simulink model "CCACC_DESIGN"  (R2023b)
settings: Solver=VariableStepAuto  StartTime=0.0  StopTime=200  RelTol=1e-3
values from neighbouring files (symbols this model uses):
  plant_den = [1084 17]    [CCACCDESIGN.m]
  plant_num = 1    [CCACCDESIGN.m]
  V_set_speed = str2double(answer)    [CCACCDESIGN.m]
undefined symbols (not defined in the file or in its folder): sigbuilder_block
libraries: slpidlib x1
settings Model: Creator=ADEL  LastModifiedBy=ADEL

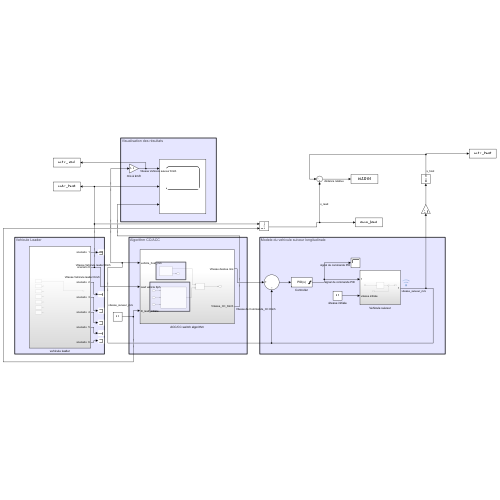
[thumbnail: Simulink's stored preview of the top-level diagram]
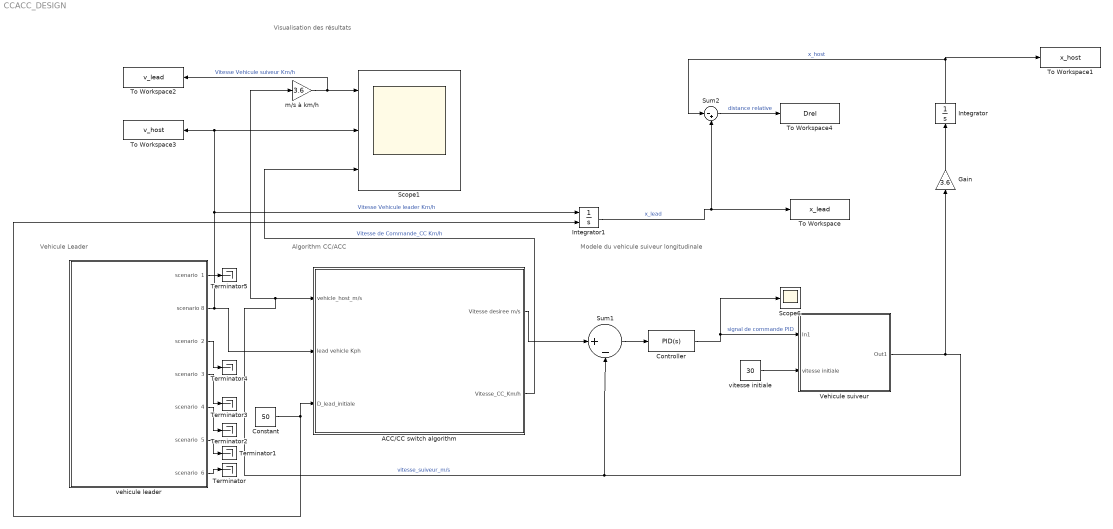
== system CCACC_DESIGN ==
  note: Visualisation des résultats
  note: Vehicule Leader
  note: Algorithm CC/ACC
  note: Modele du vehicule suiveur longitudinale
  ACC/CC switch algorithm : Subsystem
  Constant : Constant  Value=50
  Controller : slpidlib/PID Controller  Controller=PID  Form=Parallel  TimeDomain=Continuous-time  UseExternalTs=off  SampleTime=-1  IntegratorMethod=Forward Euler  FilterMethod=Forward Euler  ControllerParametersSource=internal  P=142.14884257668  I=6.71648983660147  UseKiTs=off  D=262.976834722354  N=0.25  UseFilter=on  TunerSelectOption=Transfer Function Based (PID Tuner App)  InitialConditionSource=internal  InitialConditionForIntegrator=0  InitialConditionForFilter=0  DifferentiatorICPrevScaledInput=0  ExternalReset=none  TrackingMode=off  Kt=1  LimitOutput=on  SatLimitsSource=internal  UpperSaturationLimit=4600  LowerSaturationLimit=-4600  LinearizeAsGain=on  AntiWindupMode=none  Kb=1  LimitIntegrator=off  UpperIntegratorSaturationLimit=inf  LowerIntegratorSaturationLimit=-inf  POutMin=[]  POutMax=[]  IOutMin=[]  IOutMax=[]  DOutMin=[]  DOutMax=[]  NOutMin=[]  NOutMax=[]  SumOutMin=[]  SumOutMax=[]  SaturationOutMin=[]  SaturationOutMax=[]  PParamMin=[]  PParamMax=[]  IParamMin=[]  IParamMax=[]  DParamMin=[]  DParamMax=[]  NParamMin=[]  NParamMax=[]  KbParamMin=[]  KbParamMax=[]  KtParamMin=[]  KtParamMax=[]  KbOutMin=[]  KbOutMax=[]  KtOutMin=[]  KtOutMax=[]  IntegratorOutMin=[]  IntegratorOutMax=[]  FilterOutMin=[]  FilterOutMax=[]  SumI1OutMin=[]  SumI1OutMax=[]  SumI2OutMin=[]  SumI2OutMax=[]  SumI3OutMin=[]  SumI3OutMax=[]  SumI4OutMin=[]  SumI4OutMax=[]  SumDOutMin=[]  SumDOutMax=[]  DifferentiatorOutMin=[]  DifferentiatorOutMax=[]  FilterDiffOutCoefMin=[]  FilterDiffOutCoefMax=[]  ReciprocalOutMin=[]  ReciprocalOutMax=[]  SumDenOutMin=[]  SumDenOutMax=[]  SumNumOutMin=[]  SumNumOutMax=[]  DivideOutMin=[]  DivideOutMax=[]  UdiffTsProdOutMin=[]  UdiffTsProdOutMax=[]  NTsProdOutMin=[]  NTsProdOutMax=[]  UintegralTsProdOutMin=[]  UintegralTsProdOutMax=[]  UngainTsProdOutMin=[]  UngainTsProdOutMax=[]  ClampingZeroOutDataTypeStr=Inherit: Inherit via back propagation  ClampingZeroOutMin=[]  ClampingZeroOutMax=[]  FilterDenConstantOutDataTypeStr=Inherit: Inherit via back propagation  FilterDenConstantOutMin=[]  FilterDenConstantOutMax=[]  PCopyOutDataTypeStr=Inherit: Inherit via back propagation  PCopyOutMin=[]  PCopyOutMax=[]  NCopyOutDataTypeStr=Inherit: Inherit via back propagation  NCopyOutMin=[]  NCopyOutMax=[]  IntegratorContinuousStateAttributes=''  IntegratorStateMustResolveToSignalObject=off  IntegratorRTWStateStorageClass=Auto  FilterContinuousStateAttributes=''  FilterStateMustResolveToSignalObject=off  FilterRTWStateStorageClass=Auto  ParallelPVariant=InternalParameters  IdealPVariant=Disabled  IVariant=InternalParameters  DVariant=InternalParameters  IntegratorVariant=Continuous  SatVariant=Enabled  AWVariant=Passthrough  PCopyVariant=Disabled  TRVariant=Disabled  FdbkBlocksVariant=Forward  IdealPFdbkVariant=Disabled  SatFdbkVariant=Disabled  DerivativeFilterVariant=ContFilter  NVariant=InternalParameters  NCopyVariant=Disabled  FilterICVariant=InternalICsFilter  IntegratorICVariant=InternalICs  ExternalResetVariant=Disabled  TRSumVariant=Passthrough  SumFdbkVariant=Disabled  SumVariant=Sum_PID  TsampFilterVariant=InternalTs  TsampNgainVariant=Passthrough  TsampIntegralVariant=Disabled_SignalSpec  ExternalSaturationOutDataTypeStr=Inherit: Same as second input
  Gain : Gain  Gain=3.6
  Integrator : Integrator
  Integrator1 : Integrator  InitialConditionSource=external  InitialCondition=50
  Scope1 : Scope  NumInputPorts=3
  Scope6 : Scope
  Sum1 : Sum  Inputs=|+-
  Sum2 : Sum  Inputs=|-+
  Terminator{,1..5} (6 alike) : Terminator
  To Workspace : ToWorkspace  VariableName=x_lead  SaveFormat=Structure With Time  SampleTime=-1
  To Workspace1 : ToWorkspace  VariableName=x_host  SaveFormat=Structure With Time  SampleTime=-1
  To Workspace2 : ToWorkspace  VariableName=v_lead  SaveFormat=Structure With Time  SampleTime=-1
  To Workspace3 : ToWorkspace  VariableName=v_host  SaveFormat=Structure With Time  SampleTime=-1
  To Workspace4 : ToWorkspace  VariableName=Drel  SaveFormat=Structure With Time  SampleTime=-1
  Vehicule suiveur : Subsystem
  m/s à km/h : Gain  Gain=3.6
  vehicule leader : Subsystem
  vitesse initiale : Constant  Value=30
  wires:
  Gain/1 -> Integrator/1
  vehicule leader/3(scenario  2) -> Terminator4/1
  Constant/1 -> ACC/CC switch algorithm/3(D_lead_initiale), Integrator1/2
  vehicule leader/4(scenario  3) -> Terminator3/1
  vitesse initiale/1 -> Vehicule suiveur/2(vitesse initiale)
  vehicule leader/7(scenario  6) -> Terminator/1
  Sum2/1 -> To Workspace4/1  "distance relative"
  Controller/1 -> Scope6/1, Vehicule suiveur/1(In1)  "signal de commande PID"
  vehicule leader/1(scenario  1) -> Terminator5/1
  Integrator/1 -> To Workspace1/1, Sum2/1  "x_host"
  vehicule leader/5(scenario  4) -> Terminator2/1
  Vehicule suiveur/1(Out1) -> ACC/CC switch algorithm/1(vehicle_host_m/s), m/s à km/h/1, Sum1/2, Gain/1  "vitesse_suiveur_m/s"
  vehicule leader/2(scenario 8) -> To Workspace3/1, Scope1/2, Integrator1/1, ACC/CC switch algorithm/2(lead vehicle Kph)  "Vitesse Vehicule leader Km/h"
  vehicule leader/6(scenario  5) -> Terminator1/1
  ACC/CC switch algorithm/2(Vitesse_CC_Km/h) -> Scope1/3  "Vitesse de Commande_CC Km/h"
  m/s à km/h/1 -> To Workspace2/1, Scope1/1  "Vitesse Vehicule suiveur Km/h"
  Integrator1/1 -> Sum2/2, To Workspace/1  "x_lead"
  Sum1/1 -> Controller/1
  ACC/CC switch algorithm/1(Vitesse desiree m/s) -> Sum1/1

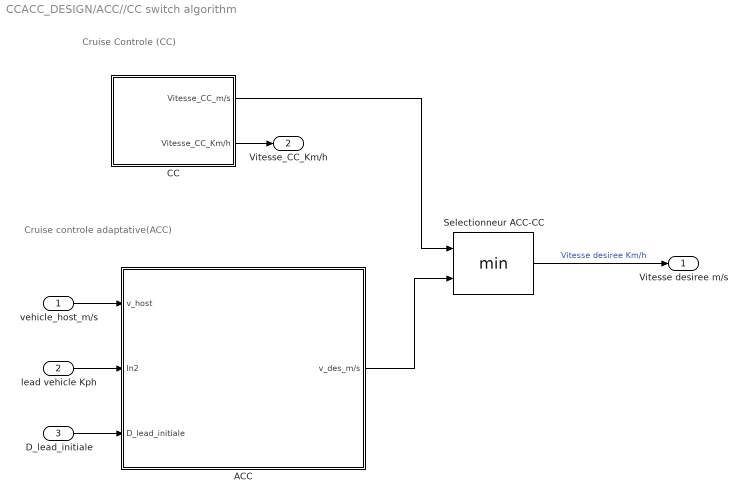
== system CCACC_DESIGN/ACC//CC switch algorithm ==
  note: Cruise controle adaptative(ACC)
  note: Cruise Controle (CC)
  vehicle_host_m/s : Inport
  lead vehicle Kph : Inport  Port=2
  D_lead_initiale : Inport  Port=3
  ACC : Subsystem
  CC : Subsystem
  Selectionneur ACC-CC : MinMax  Inputs=2
  Vitesse desiree m/s : Outport
  Vitesse_CC_Km/h : Outport  Port=2
  wires:
  CC/1(Vitesse_CC_m/s) -> Selectionneur ACC-CC/1
  vehicle_host_m/s/1 -> ACC/1(v_host)
  lead vehicle Kph/1 -> ACC/2(In2)
  ACC/1(v_des_m/s) -> Selectionneur ACC-CC/2
  CC/2(Vitesse_CC_Km/h) -> Vitesse_CC_Km/h/1
  Selectionneur ACC-CC/1 -> Vitesse desiree m/s/1  "Vitesse desiree Km/h"
  D_lead_initiale/1 -> ACC/3(D_lead_initiale)

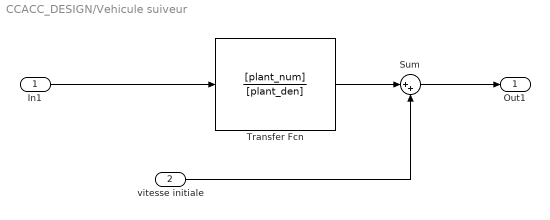
== system CCACC_DESIGN/Vehicule suiveur ==
  In1 : Inport
  vitesse initiale : Inport  Port=2
  Sum : Sum  Inputs=|++
  Transfer Fcn : TransferFcn  Numerator=[plant_num]  Denominator=[plant_den]
  Out1 : Outport
  wires:
  In1/1 -> Transfer Fcn/1
  Transfer Fcn/1 -> Sum/1
  vitesse initiale/1 -> Sum/2
  Sum/1 -> Out1/1

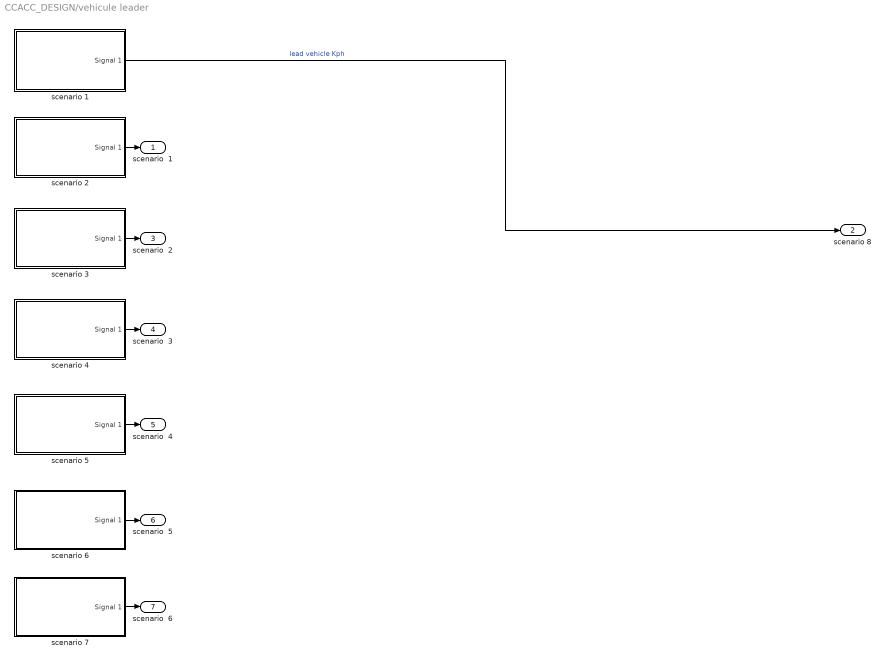
== system CCACC_DESIGN/vehicule leader ==
  scenario 1 : Subsystem  Tag=STV Subsys  LoadFcn=sigbuilder_block('load');  StartFcn=sigbuilder_block('start');  StopFcn=sigbuilder_block('stop');  ClipboardFcn=sigbuilder_block('clipboard');  mask(Sigbuilder block){tuvar=[0:10]}
      mask help: Simulink:masks:SigbuilderBlock_MD
      mask init:
      | if ~strcmp(get_param(bdroot(gcbh),'SimulationStatus'),'stopped') tuvar = sigbuilder_block('maskInit'); end
      settings: CopyFcn=sigbuilder_block('copy');  DeleteFcn=sigbuilder_block('delete');  ModelCloseFcn=sigbuilder_block('modelClose');  PreSaveFcn=sigbuilder_block('preSave');  PauseFcn=sigbuilder_block('pause');  ContinueFcn=sigbuilder_block('continue');  NameChangeFcn=sigbuilder_block('namechange');  OpenFcn=sigbuilder_block('open',[6 6 1012.5 506.25 ]);  CloseFcn=sigbuilder_block('close');
      mask Display: plot(0, 0, 100, 100,[2, 2, 32, 32, 2], [68, 8, 8, 68, 68],[32, 2], [38, 38], [32, 19, 2],[53, 60, 44], [32, 17, 17, 2],[16, 16, 31, 31]);txt = getActiveGroup(gcbh);text(2, 100, txt,'verticalAlignment', 'top');
  scenario 2 : Subsystem  Tag=STV Subsys  LoadFcn=sigbuilder_block('load');  StartFcn=sigbuilder_block('start');  StopFcn=sigbuilder_block('stop');  ClipboardFcn=sigbuilder_block('clipboard');  mask(Sigbuilder block){tuvar=[0:10]}
      mask help: Simulink:masks:SigbuilderBlock_MD
      mask init:
      | if ~strcmp(get_param(bdroot(gcbh),'SimulationStatus'),'stopped') tuvar = sigbuilder_block('maskInit'); end
      settings: CopyFcn=sigbuilder_block('copy');  DeleteFcn=sigbuilder_block('delete');  ModelCloseFcn=sigbuilder_block('modelClose');  PreSaveFcn=sigbuilder_block('preSave');  PauseFcn=sigbuilder_block('pause');  ContinueFcn=sigbuilder_block('continue');  NameChangeFcn=sigbuilder_block('namechange');  OpenFcn=sigbuilder_block('open',[34.8 6 766.8 506.25 ]);  CloseFcn=sigbuilder_block('close');
      mask Display: plot(0, 0, 100, 100,[2, 2, 32, 32, 2], [68, 8, 8, 68, 68],[32, 2], [38, 38], [32, 19, 2],[53, 60, 44], [32, 17, 17, 2],[16, 16, 31, 31]);txt = getActiveGroup(gcbh);text(2, 100, txt,'verticalAlignment', 'top');
  scenario 3 : Subsystem  Tag=STV Subsys  LoadFcn=sigbuilder_block('load');  StartFcn=sigbuilder_block('start');  StopFcn=sigbuilder_block('stop');  ClipboardFcn=sigbuilder_block('clipboard');  mask(Sigbuilder block){tuvar=[0:10]}
      mask help: Simulink:masks:SigbuilderBlock_MD
      mask init:
      | if ~strcmp(get_param(bdroot(gcbh),'SimulationStatus'),'stopped') tuvar = sigbuilder_block('maskInit'); end
      settings: CopyFcn=sigbuilder_block('copy');  DeleteFcn=sigbuilder_block('delete');  ModelCloseFcn=sigbuilder_block('modelClose');  PreSaveFcn=sigbuilder_block('preSave');  PauseFcn=sigbuilder_block('pause');  ContinueFcn=sigbuilder_block('continue');  NameChangeFcn=sigbuilder_block('namechange');  OpenFcn=sigbuilder_block('open',[34.8 6 766.8 506.25 ]);  CloseFcn=sigbuilder_block('close');
      mask Display: plot(0, 0, 100, 100,[2, 2, 32, 32, 2], [68, 8, 8, 68, 68],[32, 2], [38, 38], [32, 19, 2],[53, 60, 44], [32, 17, 17, 2],[16, 16, 31, 31]);txt = getActiveGroup(gcbh);text(2, 100, txt,'verticalAlignment', 'top');
  scenario 4 : Subsystem  Tag=STV Subsys  LoadFcn=sigbuilder_block('load');  StartFcn=sigbuilder_block('start');  StopFcn=sigbuilder_block('stop');  ClipboardFcn=sigbuilder_block('clipboard');  mask(Sigbuilder block){tuvar=[0:10]}
      mask help: Simulink:masks:SigbuilderBlock_MD
      mask init:
      | if ~strcmp(get_param(bdroot(gcbh),'SimulationStatus'),'stopped') tuvar = sigbuilder_block('maskInit'); end
      settings: CopyFcn=sigbuilder_block('copy');  DeleteFcn=sigbuilder_block('delete');  ModelCloseFcn=sigbuilder_block('modelClose');  PreSaveFcn=sigbuilder_block('preSave');  PauseFcn=sigbuilder_block('pause');  ContinueFcn=sigbuilder_block('continue');  NameChangeFcn=sigbuilder_block('namechange');  OpenFcn=sigbuilder_block('open',[34.8 6 766.8 506.25 ]);  CloseFcn=sigbuilder_block('close');
      mask Display: plot(0, 0, 100, 100,[2, 2, 32, 32, 2], [68, 8, 8, 68, 68],[32, 2], [38, 38], [32, 19, 2],[53, 60, 44], [32, 17, 17, 2],[16, 16, 31, 31]);txt = getActiveGroup(gcbh);text(2, 100, txt,'verticalAlignment', 'top');
  scenario 5 : Subsystem  Tag=STV Subsys  LoadFcn=sigbuilder_block('load');  StartFcn=sigbuilder_block('start');  StopFcn=sigbuilder_block('stop');  ClipboardFcn=sigbuilder_block('clipboard');  mask(Sigbuilder block){tuvar=[0:10]}
      mask help: Simulink:masks:SigbuilderBlock_MD
      mask init:
      | if ~strcmp(get_param(bdroot(gcbh),'SimulationStatus'),'stopped') tuvar = sigbuilder_block('maskInit'); end
      settings: CopyFcn=sigbuilder_block('copy');  DeleteFcn=sigbuilder_block('delete');  ModelCloseFcn=sigbuilder_block('modelClose');  PreSaveFcn=sigbuilder_block('preSave');  PauseFcn=sigbuilder_block('pause');  ContinueFcn=sigbuilder_block('continue');  NameChangeFcn=sigbuilder_block('namechange');  OpenFcn=sigbuilder_block('open',[34.8 6 766.8 506.25 ]);  CloseFcn=sigbuilder_block('close');
      mask Display: plot(0, 0, 100, 100,[2, 2, 32, 32, 2], [68, 8, 8, 68, 68],[32, 2], [38, 38], [32, 19, 2],[53, 60, 44], [32, 17, 17, 2],[16, 16, 31, 31]);txt = getActiveGroup(gcbh);text(2, 100, txt,'verticalAlignment', 'top');
  scenario 6 : Subsystem  Tag=STV Subsys  LoadFcn=sigbuilder_block('load');  StartFcn=sigbuilder_block('start');  StopFcn=sigbuilder_block('stop');  ClipboardFcn=sigbuilder_block('clipboard');  mask(Sigbuilder block){tuvar=[0:10]}
      mask help: Simulink:masks:SigbuilderBlock_MD
      mask init:
      | if ~strcmp(get_param(bdroot(gcbh),'SimulationStatus'),'stopped') tuvar = sigbuilder_block('maskInit'); end
      settings: CopyFcn=sigbuilder_block('copy');  DeleteFcn=sigbuilder_block('delete');  ModelCloseFcn=sigbuilder_block('modelClose');  PreSaveFcn=sigbuilder_block('preSave');  PauseFcn=sigbuilder_block('pause');  ContinueFcn=sigbuilder_block('continue');  NameChangeFcn=sigbuilder_block('namechange');  OpenFcn=sigbuilder_block('open',[34.8 6 766.8 506.25 ]);  CloseFcn=sigbuilder_block('close');
      mask Display: plot(0, 0, 100, 100,[2, 2, 32, 32, 2], [68, 8, 8, 68, 68],[32, 2], [38, 38], [32, 19, 2],[53, 60, 44], [32, 17, 17, 2],[16, 16, 31, 31]);txt = getActiveGroup(gcbh);text(2, 100, txt,'verticalAlignment', 'top');
  scenario 7 : Subsystem  Tag=STV Subsys  LoadFcn=sigbuilder_block('load');  StartFcn=sigbuilder_block('start');  StopFcn=sigbuilder_block('stop');  ClipboardFcn=sigbuilder_block('clipboard');  mask(Sigbuilder block){tuvar=[0:10]}
      mask help: Simulink:masks:SigbuilderBlock_MD
      mask init:
      | if ~strcmp(get_param(bdroot(gcbh),'SimulationStatus'),'stopped') tuvar = sigbuilder_block('maskInit'); end
      settings: CopyFcn=sigbuilder_block('copy');  DeleteFcn=sigbuilder_block('delete');  ModelCloseFcn=sigbuilder_block('modelClose');  PreSaveFcn=sigbuilder_block('preSave');  PauseFcn=sigbuilder_block('pause');  ContinueFcn=sigbuilder_block('continue');  NameChangeFcn=sigbuilder_block('namechange');  OpenFcn=sigbuilder_block('open',[6 6 1012.5 506.25 ]);  CloseFcn=sigbuilder_block('close');
      mask Display: plot(0, 0, 100, 100,[2, 2, 32, 32, 2], [68, 8, 8, 68, 68],[32, 2], [38, 38], [32, 19, 2],[53, 60, 44], [32, 17, 17, 2],[16, 16, 31, 31]);txt = getActiveGroup(gcbh);text(2, 100, txt,'verticalAlignment', 'top');
  scenario  1 : Outport
  scenario 8 : Outport  Port=2
  scenario  2 : Outport  Port=3
  scenario  3 : Outport  Port=4
  scenario  4 : Outport  Port=5
  scenario  5 : Outport  Port=6
  scenario  6 : Outport  Port=7
  wires:
  scenario 4/1(Signal 1) -> scenario  3/1
  scenario 3/1(Signal 1) -> scenario  2/1
  scenario 1/1(Signal 1) -> scenario 8/1  "lead vehicle Kph"
  scenario 2/1(Signal 1) -> scenario  1/1
  scenario 7/1(Signal 1) -> scenario  6/1
  scenario 5/1(Signal 1) -> scenario  4/1
  scenario 6/1(Signal 1) -> scenario  5/1

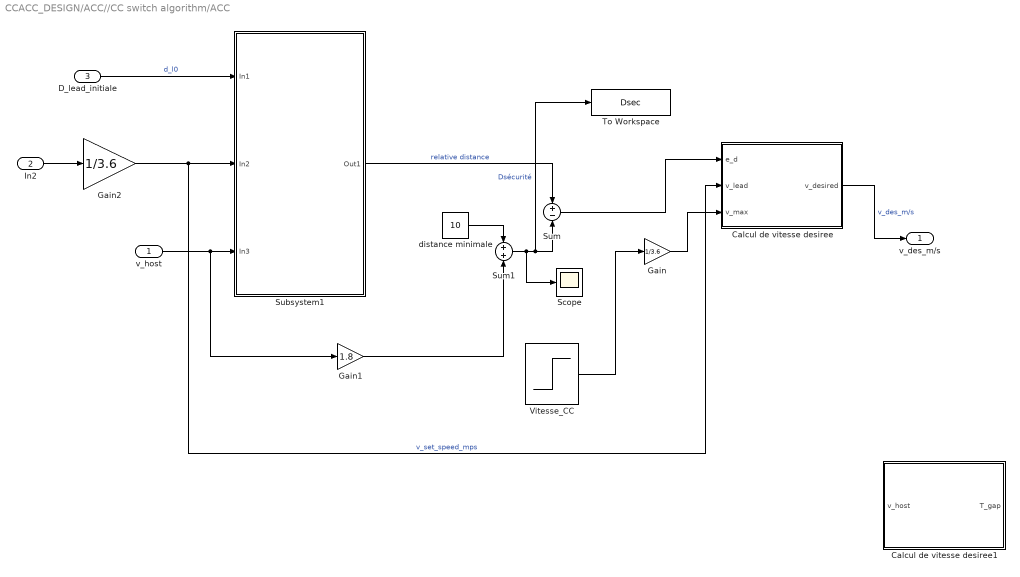
== system CCACC_DESIGN/ACC//CC switch algorithm/ACC ==
  v_host : Inport
  In2 : Inport  Port=2
  D_lead_initiale : Inport  Port=3
  Calcul de vitesse desiree : MATLAB Function  TreatAsAtomicUnit=on
  Calcul de vitesse desiree1 : MATLAB Function  TreatAsAtomicUnit=on
  Gain : Gain  Gain=1/3.6
  Gain1 : Gain  Gain=1.8
  Gain2 : Gain  Gain=1/3.6
  Scope : Scope
  Subsystem1 : Subsystem
  Sum : Sum  Inputs=+-
  Sum1 : Sum
  To Workspace : ToWorkspace  VariableName=Dsec  SaveFormat=Structure With Time  SampleTime=-1
  Vitesse_CC : Step  After=V_set_speed  SampleTime=0
  distance minimale : Constant  Value=10
  v_des_m/s : Outport
  wires:
  v_host/1 -> Gain1/1, Subsystem1/3(In3)
  Gain2/1 -> Subsystem1/2(In2), Calcul de vitesse desiree/2(v_lead)  "v_set_speed_mps"
  In2/1 -> Gain2/1
  D_lead_initiale/1 -> Subsystem1/1(In1)  "d_l0"
  Subsystem1/1(Out1) -> Sum/1  "relative distance"
  Sum/1 -> Calcul de vitesse desiree/1(e_d)
  Vitesse_CC/1 -> Gain/1
  Gain/1 -> Calcul de vitesse desiree/3(v_max)
  Calcul de vitesse desiree/1(v_desired) -> v_des_m/s/1  "v_des_m/s"
  Sum1/1 -> Scope/1, To Workspace/1, Sum/2  "Dsécurité"
  distance minimale/1 -> Sum1/1
  Gain1/1 -> Sum1/2

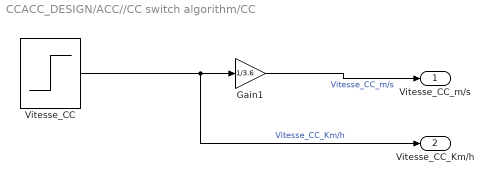
== system CCACC_DESIGN/ACC//CC switch algorithm/CC ==
  Gain1 : Gain  Gain=1/3.6
  Vitesse_CC : Step  After=V_set_speed  SampleTime=0
  Vitesse_CC_m/s : Outport
  Vitesse_CC_Km/h : Outport  Port=2
  wires:
  Vitesse_CC/1 -> Vitesse_CC_Km/h/1, Gain1/1  "Vitesse_CC_Km/h"
  Gain1/1 -> Vitesse_CC_m/s/1  "Vitesse_CC_m/s"

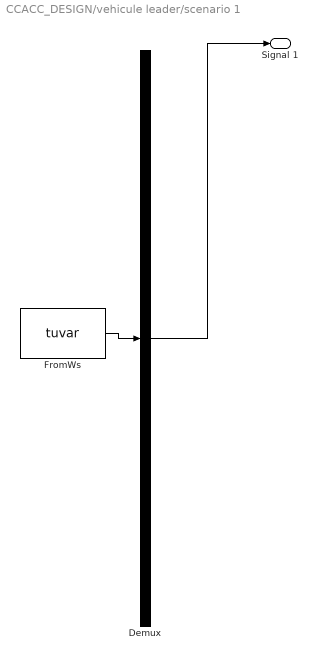
== system CCACC_DESIGN/vehicule leader/scenario 1 ==
  Demux : Demux  Tag=STV Demux  Outputs=1
      settings: DisplayOption=none
  FromWs : FromWorkspace  Tag=STV FromWs  VariableName=tuvar
      SigBuilderData=|
      | common.afterFinalStr = 'Extrapolate'
      | common.sampleTime = 0
      | dataSet.timeRange = [0 300]
      | dataSet.name = '1'
      | sbobj.Groups.Name = '1'
      | sbobj.Groups.Signals.Name = 'Signal 1'
      | sbobj.Groups.Signals.XData = [0 100 114 300]
      | sbobj.Groups.Signals.YData = [80 80 120 120]
      | sbobj.Groups.TimeRange = [0 300]
  Signal 1 : Outport  Tag=STV Outport
  wires:
  Demux/1 -> Signal 1/1
  FromWs/1 -> Demux/1

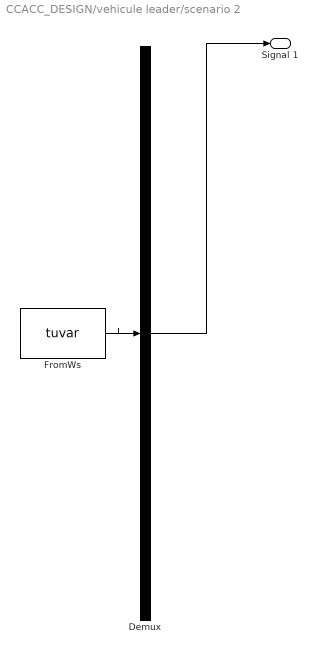
== system CCACC_DESIGN/vehicule leader/scenario 2 ==
  Demux : Demux  Tag=STV Demux  Outputs=1
      settings: DisplayOption=none
  FromWs : FromWorkspace  Tag=STV FromWs  VariableName=tuvar
      SigBuilderData=|
      | common.afterFinalStr = 'Extrapolate'
      | common.sampleTime = 0
      | dataSet.timeRange = [0 300]
      | dataSet.name = '1'
      | sbobj.Groups.Name = '1'
      | sbobj.Groups.Signals.Name = 'Signal 1'
      | sbobj.Groups.Signals.XData = [0 300]
      | sbobj.Groups.Signals.YData = [120 120]
      | sbobj.Groups.TimeRange = [0 300]
  Signal 1 : Outport  Tag=STV Outport
  wires:
  Demux/1 -> Signal 1/1
  FromWs/1 -> Demux/1

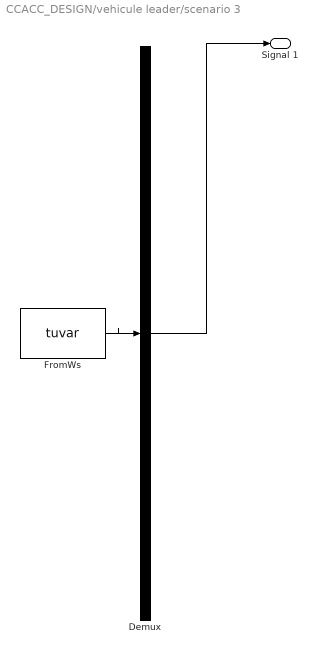
== system CCACC_DESIGN/vehicule leader/scenario 3 ==
  Demux : Demux  Tag=STV Demux  Outputs=1
      settings: DisplayOption=none
  FromWs : FromWorkspace  Tag=STV FromWs  VariableName=tuvar
      SigBuilderData=|
      | common.afterFinalStr = 'Extrapolate'
      | common.sampleTime = 0
      | dataSet.timeRange = [0 300]
      | dataSet.name = '1'
      | sbobj.Groups.Name = '1'
      | sbobj.Groups.Signals.Name = 'Signal 1'
      | sbobj.Groups.Signals.XData = [0 38 50 53.5 300]
      | sbobj.Groups.Signals.YData = [0 110 110 0 0]
      | sbobj.Groups.TimeRange = [0 300]
  Signal 1 : Outport  Tag=STV Outport
  wires:
  Demux/1 -> Signal 1/1
  FromWs/1 -> Demux/1

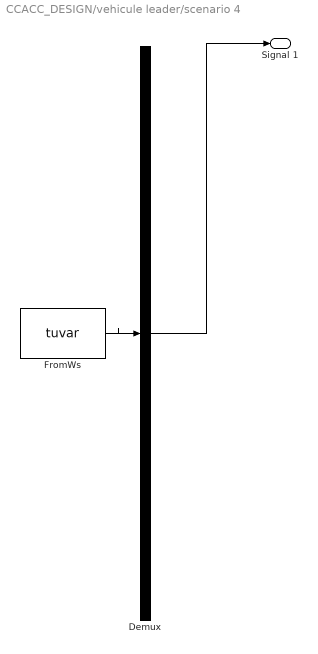
== system CCACC_DESIGN/vehicule leader/scenario 4 ==
  Demux : Demux  Tag=STV Demux  Outputs=1
      settings: DisplayOption=none
  FromWs : FromWorkspace  Tag=STV FromWs  VariableName=tuvar
      SigBuilderData=|
      | common.afterFinalStr = 'Extrapolate'
      | common.sampleTime = 0
      | dataSet.timeRange = [0 300]
      | dataSet.name = '1'
      | sbobj.Groups.Name = '1'
      | sbobj.Groups.Signals.Name = 'Signal 1'
      | sbobj.Groups.Signals.XData = [0 30 40 43 300]
      | sbobj.Groups.Signals.YData = [0 90 90 0 0]
      | sbobj.Groups.TimeRange = [0 300]
  Signal 1 : Outport  Tag=STV Outport
  wires:
  Demux/1 -> Signal 1/1
  FromWs/1 -> Demux/1

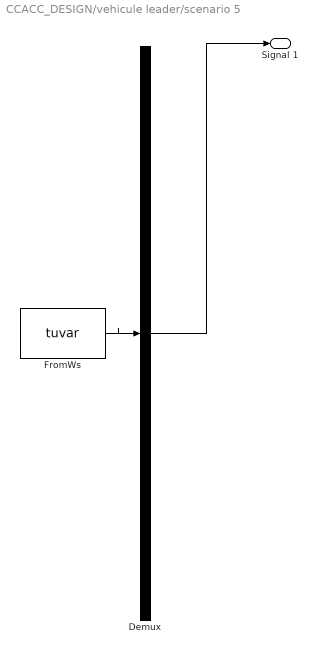
== system CCACC_DESIGN/vehicule leader/scenario 5 ==
  Demux : Demux  Tag=STV Demux  Outputs=1
      settings: DisplayOption=none
  FromWs : FromWorkspace  Tag=STV FromWs  VariableName=tuvar
      SigBuilderData=|
      | common.afterFinalStr = 'Extrapolate'
      | common.sampleTime = 0
      | dataSet.timeRange = [0 300]
      | dataSet.name = '1'
      | sbobj.Groups.Name = '1'
      | sbobj.Groups.Signals.Name = 'Signal 1'
      | sbobj.Groups.Signals.XData = [0 47 60 63.5 63.5 300]
      | sbobj.Groups.Signals.YData = [0 140 140 79.5 55 53.5]
      | sbobj.Groups.TimeRange = [0 300]
  Signal 1 : Outport  Tag=STV Outport
  wires:
  Demux/1 -> Signal 1/1
  FromWs/1 -> Demux/1

== system CCACC_DESIGN/vehicule leader/scenario 6 ==
  Demux : Demux  Tag=STV Demux  Outputs=1
      settings: DisplayOption=none
  FromWs : FromWorkspace  Tag=STV FromWs  VariableName=tuvar
      SigBuilderData=|
      | common.afterFinalStr = 'Extrapolate'
      | common.sampleTime = 0
      | dataSet.timeRange = [0 300]
      | dataSet.name = '1'
      | sbobj.Groups.Name = '1'
      | sbobj.Groups.Signals.Name = 'Signal 1'
      | sbobj.Groups.Signals.XData = [0 300]
      | sbobj.Groups.Signals.YData = [80.005 80]
      | sbobj.Groups.TimeRange = [0 300]
  Signal 1 : Outport  Tag=STV Outport
  wires:
  Demux/1 -> Signal 1/1
  FromWs/1 -> Demux/1

== system CCACC_DESIGN/vehicule leader/scenario 7 ==
  Demux : Demux  Tag=STV Demux  Outputs=1
      settings: DisplayOption=none
  FromWs : FromWorkspace  Tag=STV FromWs  VariableName=tuvar
      SigBuilderData=|
      | common.afterFinalStr = 'Extrapolate'
      | common.sampleTime = 0
      | dataSet.timeRange = [0 300]
      | dataSet.name = '1'
      | sbobj.Groups.Name = '1'
      | sbobj.Groups.Signals.Name = 'Signal 1'
      | sbobj.Groups.Signals.XData = [0 13.5 17 22 24 38.5 42 47 49 63.5 67 72 74 74 300]
      | sbobj.Groups.Signals.YData = [0 0 10 10 0 0 10 10 0 0 10 10 -0.02 0 0]
      | sbobj.Groups.TimeRange = [0 300]
  Signal 1 : Outport  Tag=STV Outport
  wires:
  Demux/1 -> Signal 1/1
  FromWs/1 -> Demux/1

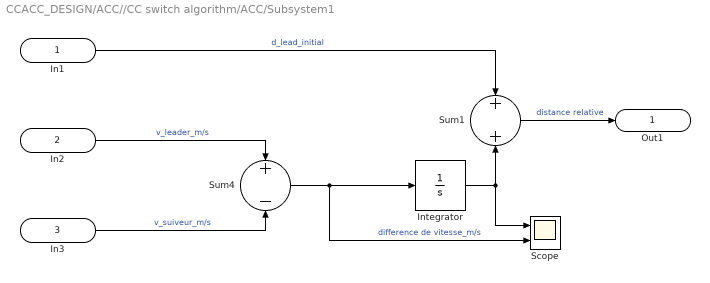
== system CCACC_DESIGN/ACC//CC switch algorithm/ACC/Subsystem1 ==
  In1 : Inport
  In2 : Inport  Port=2
  In3 : Inport  Port=3
  Integrator : Integrator
  Scope : Scope  NumInputPorts=2
  Sum1 : Sum
  Sum4 : Sum  Inputs=+-
  Out1 : Outport
  wires:
  In1/1 -> Sum1/1  "d_lead_initial"
  In2/1 -> Sum4/1  "v_leader_m/s"
  In3/1 -> Sum4/2  "v_suiveur_m/s"
  Sum4/1 -> Scope/2, Integrator/1  "difference de vitesse_m/s"
  Integrator/1 -> Scope/1, Sum1/2
  Sum1/1 -> Out1/1  "distance relative"

== matlab function CCACC_DESIGN/ACC//CC switch algorithm/ACC/Calcul de vitesse desiree1 ==
  data: T_gap output; v_host input
function T_gap = getTimeGap(v_host)
%#codegen

% This function sets a desired time gap based on velocity

if v_host <= 10
    T_gap = 1.5;
elseif v_host <= 20
    T_gap = 2;
elseif v_host <= 30
    T_gap = 3.5;
else
    T_gap = 4;
end

== matlab function CCACC_DESIGN/ACC//CC switch algorithm/ACC/Calcul de vitesse desiree ==
  data: v_desired output; e_d input; v_lead input; v_max input
function v_desired = compute_desired_velocity(e_d, v_lead, v_max)
%#codegen
% Calculates desired velocity based on distance error and lead car speed
% Inputs:
%   e_d     - Distance error (m)
%   v_lead  - Velocity of lead vehicle (m/s)
%   v_max   - Max allowed speed (m/s)
%
% Output:
%   v_desired - Desired velocity for host vehicle (m/s)

    % Proportional gain for distance error
    Kp = 0.5;

    % Adjust velocity based on distance error
    delta_v = Kp * e_d;

    % Desired velocity before bounding
    v_raw = v_lead + delta_v;

    % Bound desired velocity to not exceed limits or go negative
    v_desired = min(max(v_raw, 0), v_max);
end
